simulink model "observer"  (R2022b)
settings: Solver=VariableStepAuto  StartTime=0.0  StopTime=2  RelTol=1e-3
values from neighbouring files (symbols this model uses):
  Ad = ss_d.A    [ControllerwithDelay.m]    (also in ControllerwithDelay_LQR.m; ControllerwithDelay_PID.m; ControllerwithDelay_SS.m; DiscreteLQControl.m)
  Aobs = Ad-KDiscObe*Cd    [DiscreteObserver.m]
  Bd = ss_d.B    [ControllerwithDelay.m]    (also in ControllerwithDelay_LQR.m; ControllerwithDelay_PID.m; ControllerwithDelay_SS.m; DiscreteLQControl.m)
  Bobs = [Bd KDiscObe]    [DiscreteObserver.m]
  Cd = ss_d.C    [ControllerwithDelay.m]    (also in ControllerwithDelay_LQR.m; ControllerwithDelay_PID.m; ControllerwithDelay_SS.m; DiscreteLQControl.m)
  kDisc = place(Ad,Bd,[0.5 0.4+0.3j 0.4-0.3j])    [DiscreteObserver.m]
libraries: simulink x1
settings Model: Creator=1  LastModifiedBy=DAVID CHEN
settings ModelReferenceCC: EnableRefExpFcnMdlSchedulingChecks=on

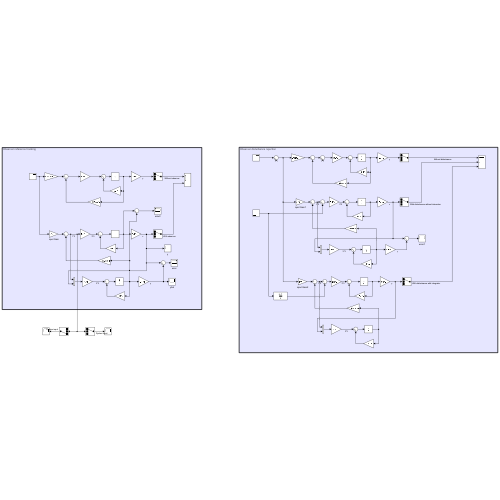
[thumbnail: Simulink's stored preview of the top-level diagram]
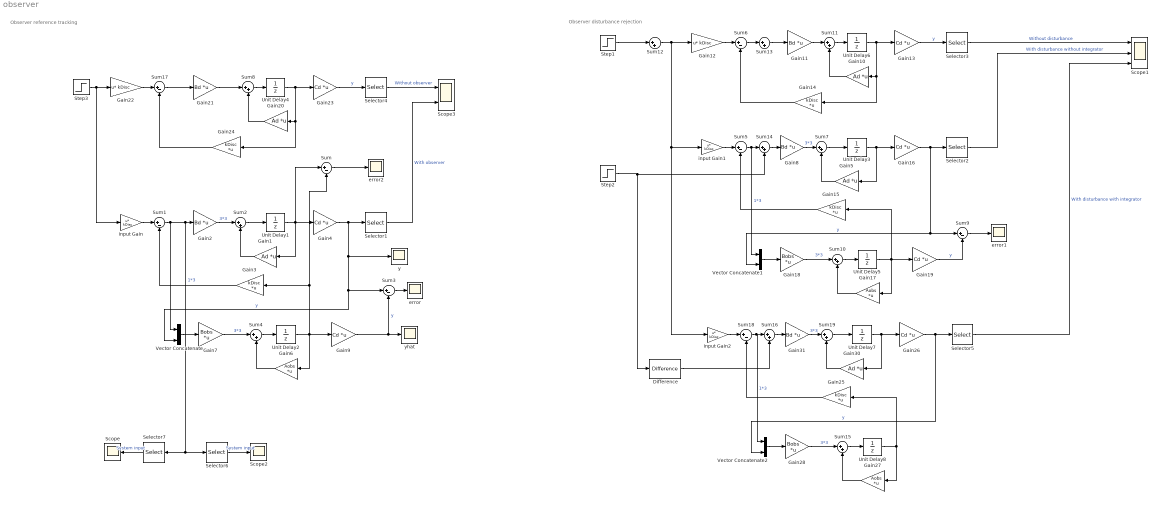
== system observer ==
  note: Observer disturbance rejection
  note: Observer reference tracking
  Difference : simulink/Discrete/Difference  ICPrevInput=0.0  OutMin=[]  OutMax=[]  OutDataType=fixdt(1, 16)  OutScaling=2^-10  DoSatur=off
  Gain{1,5,10,20,30} (5 alike) : Gain  Gain=Ad  Multiplication=Matrix(K*u)
  Gain{2,8,11,21,31} (5 alike) : Gain  Gain=Bd  Multiplication=Matrix(K*u)
  Gain12 : Gain  Gain=kDisc  Multiplication=Matrix(u*K)
  Gain{4,9,13,16,19,23,26} (7 alike) : Gain  Gain=Cd  Multiplication=Matrix(K*u)
  Gain{3,14..15,24..25} (5 alike) : Gain  Gain=kDisc  Multiplication=Matrix(K*u)
  Gain17 : Gain  Gain=Aobs  Multiplication=Matrix(K*u)
  Gain18 : Gain  Gain=Bobs  Multiplication=Matrix(K*u)
  Gain22 : Gain  Gain=kDisc  Multiplication=Matrix(u*K)
  Gain27 : Gain  Gain=Aobs  Multiplication=Matrix(K*u)
  Gain28 : Gain  Gain=Bobs  Multiplication=Matrix(K*u)
  Gain6 : Gain  Gain=Aobs  Multiplication=Matrix(K*u)
  Gain7 : Gain  Gain=Bobs  Multiplication=Matrix(K*u)
  Scope : Scope
  Scope1 : Scope  NumInputPorts=3
  Scope2 : Scope
  Scope3 : Scope  NumInputPorts=2
  Selector{1..6} (6 alike) : Selector  InputPortWidth=3  IndexOptions=Index vector (dialog)  Indices=[1]  OutputSizes=1
  Selector7 : Selector  InputPortWidth=3  IndexOptions=Index vector (dialog)  Indices=[3]  OutputSizes=1
  Step1 : Step  Time=0.1  SampleTime=0
  Step2 : Step  Time=5  SampleTime=0
  Step3 : Step  Time=0.1  SampleTime=0
  Sum{,1,3,5..6,9,17..18} (8 alike) : Sum  Inputs=|+-
  Sum{2,4,7..8,10..16,19} (12 alike) : Sum  Inputs=|++
  Unit Delay{1,3..4,6..7} (5 alike) : UnitDelay  InitialCondition=0.5  SampleTime=-1  HasFrameUpgradeWarning=on
  Unit Delay2 : UnitDelay  SampleTime=-1  HasFrameUpgradeWarning=on
  Unit Delay5 : UnitDelay  SampleTime=-1  HasFrameUpgradeWarning=on
  Unit Delay8 : UnitDelay  SampleTime=-1  HasFrameUpgradeWarning=on
  Vector Concatenate : Concatenate  Mode=Multidimensional array
  Vector Concatenate1 : Concatenate  Mode=Multidimensional array
  Vector Concatenate2 : Concatenate  Mode=Multidimensional array
  error : Scope
  error1 : Scope
  error2 : Scope
  input Gain : Gain  Gain=kDisc  Multiplication=Matrix(u*K)
  input Gain1 : Gain  Gain=kDisc  Multiplication=Matrix(u*K)
  input Gain2 : Gain  Gain=kDisc  Multiplication=Matrix(u*K)
  y : Scope
  yhat : Scope
  wires:
  Sum8/1 -> Unit Delay4/1
  Gain20/1 -> Sum8/2
  Gain21/1 -> Sum8/1
  Selector4/1 -> Scope3/1  "Without observer"
  Gain24/1 -> Sum17/2
  Sum17/1 -> Gain21/1
  Unit Delay4/1 -> Gain20/1, Gain24/1, Gain23/1
  Gain22/1 -> Sum17/1
  Gain23/1 -> Selector4/1  "y"
  Gain4/1 -> y/1, Sum3/1, Vector Concatenate/2, Selector1/1  "y"
  Sum1/1 -> Vector Concatenate/1, Selector7/1, Selector6/1, Gain2/1  "1*3"
  Step3/1 -> input Gain/1, Gain22/1
  Gain1/1 -> Sum2/2
  Unit Delay1/1 -> Sum/1, Gain1/1, Gain4/1
  Gain2/1 -> Sum2/1  "3*3"
  Sum2/1 -> Unit Delay1/1
  Selector1/1 -> Scope3/2  "With observer"
  Gain6/1 -> Sum4/2
  Sum4/1 -> Unit Delay2/1
  Unit Delay2/1 -> Sum/2, Gain3/1, Gain9/1, Gain6/1
  Gain7/1 -> Sum4/1  "3*3"
  Gain9/1 -> Sum3/2, yhat/1  "y"
  input Gain/1 -> Sum1/1
  Gain3/1 -> Sum1/2
  Vector Concatenate/1 -> Gain7/1
  Sum3/1 -> error/1
  Vector Concatenate1/1 -> Gain18/1
  Gain13/1 -> Selector3/1  "y"
  Gain14/1 -> Sum6/2
  Selector3/1 -> Scope1/1  "Without disturbance"
  Gain11/1 -> Sum11/1
  Sum11/1 -> Unit Delay6/1
  Gain15/1 -> Sum5/2
  Sum9/1 -> error1/1
  Gain8/1 -> Sum7/1  "3*3"
  Unit Delay5/1 -> Gain15/1, Gain19/1, Gain17/1
  Gain12/1 -> Sum6/1
  Gain5/1 -> Sum7/2
  Sum10/1 -> Unit Delay5/1
  Gain10/1 -> Sum11/2
  Sum7/1 -> Unit Delay3/1
  Gain18/1 -> Sum10/1  "3*3"
  Unit Delay3/1 -> Gain5/1, Gain16/1
  Gain17/1 -> Sum10/2
  Gain19/1 -> Sum9/2  "y"
  Gain16/1 -> Vector Concatenate1/2, Sum9/1, Selector2/1  "y"
  Unit Delay6/1 -> Gain10/1, Gain14/1, Gain13/1
  input Gain1/1 -> Sum5/1
  Sum5/1 -> Vector Concatenate1/1, Sum14/1  "1*3"
  Selector2/1 -> Scope1/2  "With disturbance without integrator"
  Step1/1 -> Sum12/1
  Sum12/1 -> input Gain2/1, input Gain1/1, Gain12/1
  Sum6/1 -> Sum13/1
  Sum13/1 -> Gain11/1
  Sum14/1 -> Gain8/1
  Sum16/1 -> Gain31/1
  Sum18/1 -> Vector Concatenate2/1, Sum16/1  "1*3"
  Gain26/1 -> Vector Concatenate2/2, Selector5/1  "y"
  input Gain2/1 -> Sum18/1
  Gain28/1 -> Sum15/1  "3*3"
  Gain27/1 -> Sum15/2
  Sum19/1 -> Unit Delay7/1
  Sum15/1 -> Unit Delay8/1
  Unit Delay8/1 -> Gain25/1, Gain27/1
  Gain30/1 -> Sum19/2
  Unit Delay7/1 -> Gain30/1, Gain26/1
  Vector Concatenate2/1 -> Gain28/1
  Gain31/1 -> Sum19/1  "3*3"
  Gain25/1 -> Sum18/2
  Selector5/1 -> Scope1/3  "With disturbance with integrator"
  Step2/1 -> Difference/1, Sum14/2
  Difference/1 -> Sum16/2
  Selector6/1 -> Scope2/1  "System input"
  Selector7/1 -> Scope/1  "System input"
  Sum/1 -> error2/1
